simulink library "windTurbine_ul"  (R2018b)
settings: Solver=VariableStepAuto  StartTime=0.0  StopTime=10.0  RelTol=1e-3
libraries: simulink x1, eulAng2RotMat_ul x1, filteredPIDController_ul x1
settings Model: Creator=asiddiq2  LastModifiedBy=asiddiq2

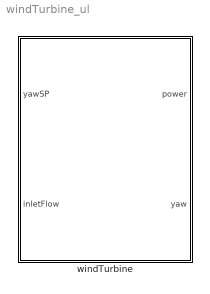
== system windTurbine_ul ==
  windTurbine : Subsystem  mask{Cp=0, rhoFluid=0, diam=0, dampCoeff=0, Izz=0, iniYaw=0, Kp=0, Ki=0, Kd=0, tau=0}
      mask prompts: Cp "Power coefficient"; rhoFluid "Fluid density"; diam "Turbine diameter"; dampCoeff "Damping coefficient"; Izz "MI"; iniYaw "Initial yaw"; Kp "Proportional gain"; Ki "Integral gain"; Kd "Derivative gain"; tau "Time constant"
      mask DialogControl Container3 Prompt: Controller

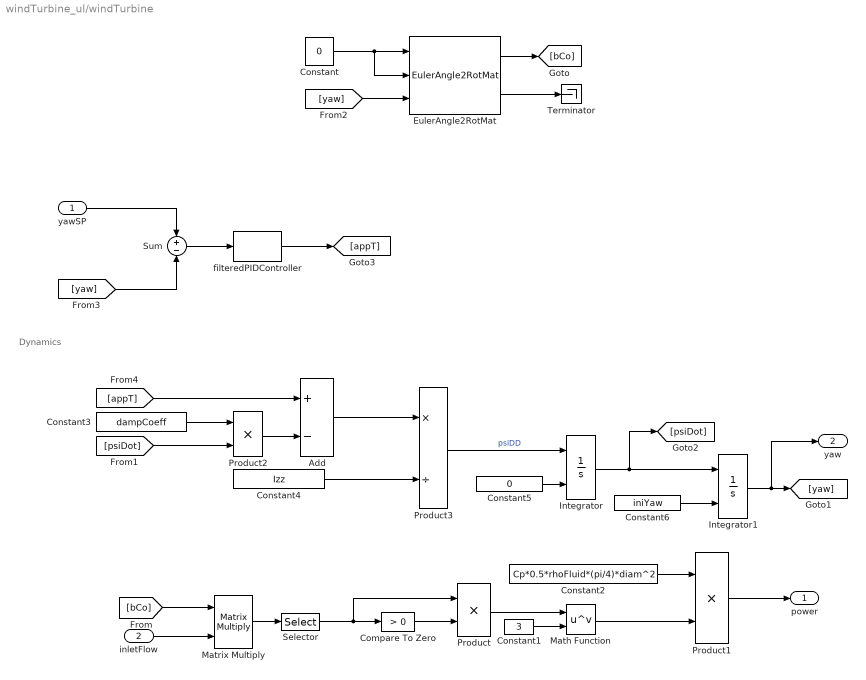
== system windTurbine_ul/windTurbine ==
  note: Dynamics
  yawSP : Inport
  inletFlow : Inport  Port=2
  Add : Sum  Inputs=+-
  Compare To Zero : simulink/Logic and Bit Operations/Compare To Zero  relop=>  OutDataTypeStr=boolean
  Constant : Constant  Value=0
  Constant1 : Constant  Value=3
  Constant2 : Constant  Value=Cp*0.5*rhoFluid*(pi/4)*diam^2
  Constant3 : Constant  Value=dampCoeff  VectorParams1D=off
  Constant4 : Constant  Value=Izz  VectorParams1D=off
  Constant5 : Constant  Value=0  VectorParams1D=off
  Constant6 : Constant  Value=iniYaw  VectorParams1D=off
  EulerAngle2RotMat : eulAng2RotMat_ul/EulerAngle2RotMat  SystemSampleTime=-1
  Integrator : Integrator  InitialConditionSource=external
  Integrator1 : Integrator  InitialConditionSource=external
  Math Function : Math  Operator=pow  SaturateOnIntegerOverflow=on
  Matrix Multiply : Product  Multiplication=Matrix(*)
  Product : Product
  Product1 : Product
  Product2 : Product
  Product3 : Product  Inputs=*/
  Selector : Selector  NumberOfDimensions=2  InputPortWidth=3  IndexOptions=Index vector (dialog),Index vector (dialog)  Indices=1,1  OutputSizes=1,1
  Sum : Sum  Inputs=+-
  Terminator : Terminator
  filteredPIDController : filteredPIDController_ul/filteredPIDController  kp=Kp  ki=Ki  kd=Kd  Value=tau
  power : Outport
  yaw : Outport  Port=2
  wires:
  Constant/1 -> EulerAngle2RotMat/2, EulerAngle2RotMat/1
  EulerAngle2RotMat/2 -> Terminator/1
  EulerAngle2RotMat/1 -> [bCo]
  [bCo] -> Matrix Multiply/1
  inletFlow/1 -> Matrix Multiply/2
  Matrix Multiply/1 -> Selector/1
  Selector/1 -> Product/1, Compare To Zero/1
  Compare To Zero/1 -> Product/2
  Product/1 -> Math Function/1
  Constant1/1 -> Math Function/2
  Math Function/1 -> Product1/2
  Constant2/1 -> Product1/1
  Product1/1 -> power/1
  [appT] -> Add/1
  Product2/1 -> Add/2
  Constant3/1 -> Product2/1
  [psiDot] -> Product2/2
  Add/1 -> Product3/1
  Constant4/1 -> Product3/2
  Product3/1 -> Integrator/1  "psiDD"
  Integrator/1 -> [psiDot], Integrator1/1
  Constant5/1 -> Integrator/2
  Constant6/1 -> Integrator1/2
  Integrator1/1 -> yaw/1, [yaw]
  [yaw] -> EulerAngle2RotMat/3
  yawSP/1 -> Sum/1
  [yaw] -> Sum/2
  Sum/1 -> filteredPIDController/1
  filteredPIDController/1 -> [appT]
